simulink model "a1ae1"  (R2022a)
settings: Solver=VariableStepAuto  StartTime=0.0  StopTime=0.1  RelTol=1e-3
settings Model: Creator=attit  LastModifiedBy=attit

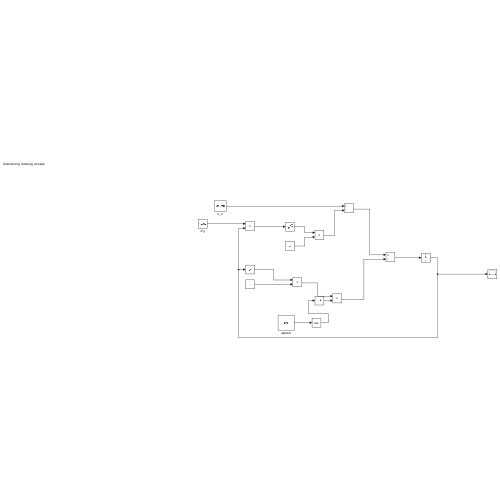
[thumbnail: Simulink's stored preview of the top-level diagram]
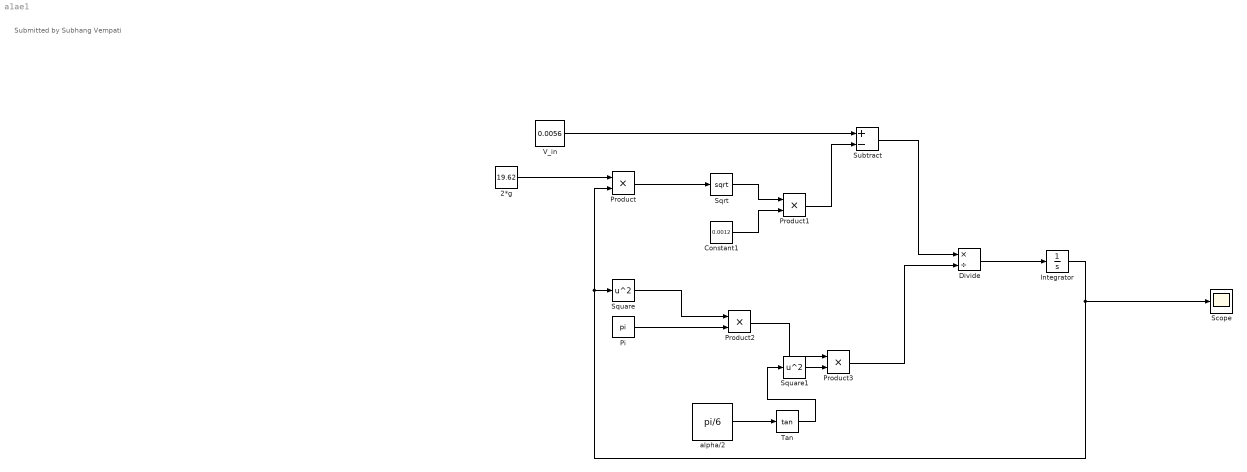
== system a1ae1 ==
  note: Submitted by Subhang Vempati
  2*g : Constant  Value=19.62
  Constant1 : Constant  Value=0.0012
  Divide : Product  Inputs=*/
  Integrator : Integrator  InitialCondition=0.0000000001
  Pi : Constant  Value=pi  OutDataTypeStr=Inherit: Inherit via back propagation
  Product{,1..3} (4 alike) : Product
  Scope : Scope
  Sqrt : Sqrt
  Square : Math  Operator=square
  Square1 : Math  Operator=square
  Subtract : Sum  Inputs=+-
  Tan : Trigonometry  Operator=tan
  V_in : Constant  Value=0.0056
  alpha/2 : Constant  Value=pi/6
  wires:
  V_in/1 -> Subtract/1
  2*g/1 -> Product/1
  Product/1 -> Sqrt/1
  Sqrt/1 -> Product1/1
  Constant1/1 -> Product1/2
  Product1/1 -> Subtract/2
  Pi/1 -> Product2/2
  Square/1 -> Product2/1
  alpha/2/1 -> Tan/1
  Product2/1 -> Product3/1
  Product3/1 -> Divide/2
  Subtract/1 -> Divide/1
  Divide/1 -> Integrator/1
  Integrator/1 -> Scope/1, Product/2, Square/1
  Tan/1 -> Square1/1
  Square1/1 -> Product3/2
